simulink model "Lab1_StateDiagram"  (R2016a)
settings: Solver=VariableStepAuto  StartTime=0.0  StopTime=100  RelTol=1e-3
settings Model: Creator=Daniel  LastModifiedBy=Daniel

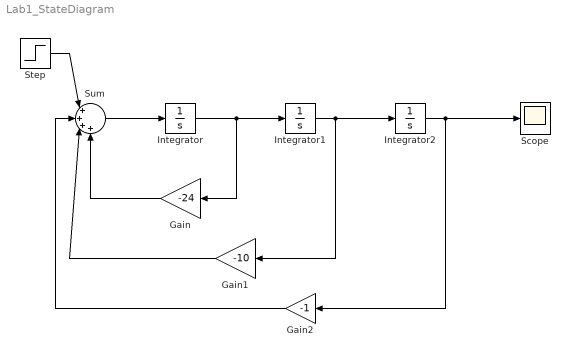
== system Lab1_StateDiagram ==
  Gain : Gain  Gain=-24
  Gain1 : Gain  Gain=-10
  Gain2 : Gain  Gain=-1
  Integrator : Integrator
  Integrator1 : Integrator
  Integrator2 : Integrator
  Scope : Scope
  Step : Step  SampleTime=0
  Sum : Sum  Inputs=|++++
  wires:
  Sum/1 -> Integrator/1
  Gain/1 -> Sum/4
  Integrator/1 -> Integrator1/1, Gain/1
  Gain1/1 -> Sum/3
  Integrator1/1 -> Integrator2/1, Gain1/1
  Gain2/1 -> Sum/2
  Integrator2/1 -> Scope/1, Gain2/1
  Step/1 -> Sum/1
